simulink model "FA2and3"  (R2022a)
settings: Solver=VariableStepAuto  StartTime=0.0  StopTime=25  RelTol=1e-3
model workspace (MAT data in the model file):
  E_thr = 1
  FA_max = 0.507853183638
  IPTG = 0
  K_Emu = 0.365971476042
  K_I = 19.9270766366
  K_M = 0.73500041743
  K_SP = 0.0154496056241
  K_h = 0.351483372423
  L0 = 0.00183809982396
  X0 = 0.102899560556
  X_max = 1.78075878444
  d_E = 0.097029794518
  d_L = 1.386
  k_E = 0.642735769035
  k_L1 = 19.0840714003
  k_L2 = 98.2931695522
  k_M = 0.431992161145
  k_X = 0.512344522231
  mu_d = 0.0112144712874
  n_Emu = 3.18736525631
  n_I = 1.01840378857
  n_L = 0.608694415816
  n_h = 1.08228942427
  tox_mumax = 0.524202832005
settings Model: Creator=tomok  LastModifiedBy=tomok
settings DataIOCC: ReturnWorkspaceOutputsName=SDOSimTest_Log

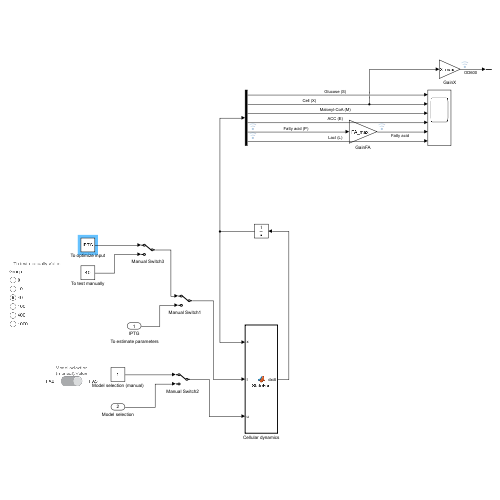
[thumbnail: Simulink's stored preview of the top-level diagram]
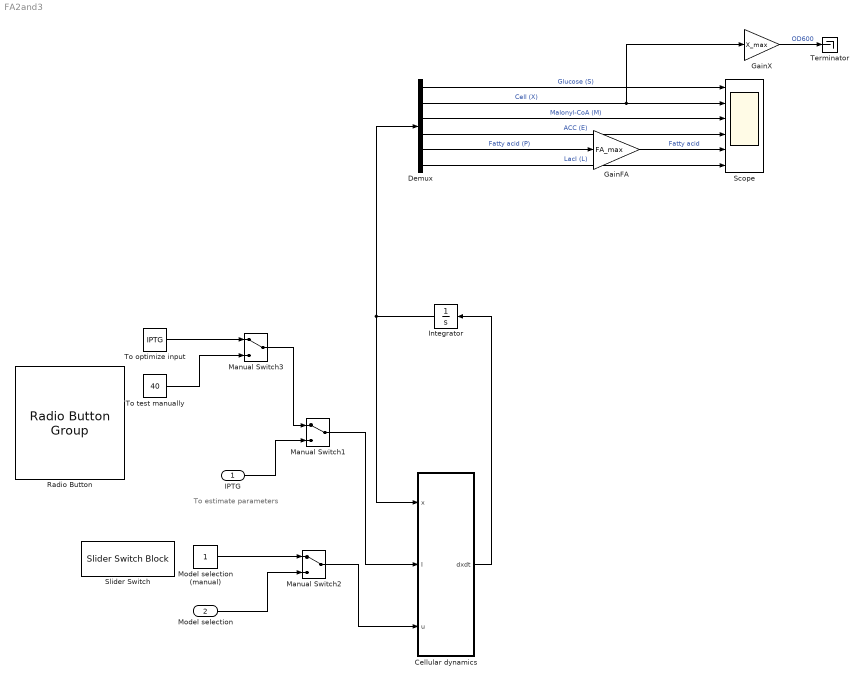
== system FA2and3 ==
  note: To estimate parameters
  IPTG : Inport
  Model selection : Inport  Port=2
  Cellular dynamics : MATLAB Function  TreatAsAtomicUnit=on
  Demux : Demux  Outputs=6
  GainFA : Gain  Gain=FA_max
  GainX : Gain  Gain=X_max
  Integrator : Integrator  InitialCondition=[1 - X0; X0; 0; 0; 0; L0]
  Manual Switch1 : ManualSwitch
  Manual Switch2 : ManualSwitch
  Manual Switch3 : ManualSwitch
  Model selection (manual) : Constant
  Radio Button : RadioButtonGroup  SelectedLabel=40  ButtonGroupName=Group
      settings: Values={{'0', '10', '40', '100', '400', '1000'}, [0 10 40 100 400 1000]}
  Scope : Scope  NumInputPorts=6
  Slider Switch : SliderSwitchBlock
      settings: Values={{'FA2', 'FA3'}, [0 1]}
  Terminator : Terminator
  To optimize input : Constant  Value=IPTG  VectorParams1D=off
  To test manually : Constant  Value=40
  wires:
  Cellular dynamics/1(dxdt) -> Integrator/1
  Integrator/1 -> Demux/1, Cellular dynamics/1(x)
  Demux/1 -> Scope/1  "Glucose (S)"
  Demux/2 -> GainX/1, Scope/2  "Cell (X)"
  Demux/3 -> Scope/3  "Malonyl-CoA (M)"
  Demux/4 -> Scope/4  "ACC (E)"
  IPTG/1 -> Manual Switch1/2
  Manual Switch1/1 -> Cellular dynamics/2(I)
  GainX/1 -> Terminator/1  "OD600"
  To test manually/1 -> Manual Switch3/2
  Demux/6 -> Scope/6  "LacI (L)"
  Demux/5 -> GainFA/1  "Fatty acid (P)"
  Model selection (manual)/1 -> Manual Switch2/1
  Manual Switch2/1 -> Cellular dynamics/3(u)
  Model selection/1 -> Manual Switch2/2
  GainFA/1 -> Scope/5  "Fatty acid"
  To optimize input/1 -> Manual Switch3/1
  Manual Switch3/1 -> Manual Switch1/1

== matlab function FA2and3/Cellular dynamics ==
  data: x input; dxdt output; I input; u input; k_X parameter; mu_d parameter; d_E parameter; k_E parameter; K_SP parameter; k_M parameter; d_L parameter; k_L1 parameter; k_L2 parameter; tox_mumax parameter; K_Emu parameter; n_Emu parameter; E_thr parameter; K_h parameter; n_h parameter; K_I parameter; n_I parameter; n_L parameter; K_M parameter
function dxdt = StateFcn(x,I,u,k_X, mu_d, d_E, k_E, K_SP, k_M, d_L, k_L1, k_L2, tox_mumax, K_Emu, n_Emu, E_thr, K_h, n_h, K_I, n_I, n_L, K_M)
%% Inputs
% I = 103;
% P(T7) response is 
% 0.2 @  40 uM
% 0.4 @ 100 uM

% u = 1; % 1 is FA3, 2 is FA2

%% Parameters
% k_X = 0.5;
% mu_d = 0.01; % cell death rate
% d_E = 0.20; % from [Xu,2020]
% k_E = 1;
% K_SP = 0.01;
% 
% % these two parameters must be the same!
% k_M = 0.5;
% 
% d_L = 1.386; % [Basu+,2005]
% k_L1 = 34.65; % d_L*25;
% k_L2 = 57.1725; % k_L1*1.65;
% % K_L = 1; % defined parameter
% 
% % ACC toxicity parameters
% tox_mumax = 0.5;
% K_Emu = 1;
% n_Emu = 4;
% E_thr = 1; % defined parameter
% K_h = 0.2; % IMPORTANT!
% n_h = 4;
% 
% % P(T7) parameters
% K_I = 10; % [uM]
% n_I = 1.2; % [-]
% n_L = 1; % [-]
% 
% % P(FR1) parameters
% % M_max = 6.43; % 26.7 [uM];
% K_M = 0.4;

k_P = k_M;
n_M = 4; % [Xu,2020]

%% State variables
S = x(1);
X = x(2);
M = x(3);
E = x(4);
% P = x(5);
L = x(6);

%% ACC toxicity
% growth slowdown
tox_mu = tox_mumax*(E^n_Emu/(K_Emu^n_Emu + E^n_Emu));

% cell health
Eex = E - E_thr;
if Eex < 0
    h = 1;
else 
    h = K_h^n_h/(Eex^n_h + K_h^n_h);
end

%% Malonyl-CoA sensor (P(FR1))
z = M^n_M/(M^n_M + K_M^n_M);

%% Reaction rates
mu = k_X*S*(1 - tox_mu);
r_X = mu*X;
r_M = k_M*E;
r_P = k_P*M;

%% ODEs
dSdt = - r_X;
dXdt = r_X - mu_d*X;

dMdt = r_M - r_P- mu*M;
dPdt = r_P*X*(S/(S + K_SP))*h;

dEdt = k_E*P_T7(L,I,K_I,n_I,n_L) - (d_E + mu)*E;
dLdt = k_L1 + u*k_L2*z - (d_L + mu)*L;

dxdt = [dSdt; dXdt; dMdt; dEdt; dPdt; dLdt;];

% lower limit of states
dxdt(x < 0 & dxdt < 0) = 0;
end
